simulink model "mux_axi"  (R2023b)
settings: Solver=FixedStepDiscrete  StartTime=0.0  StopTime=1000e-7  RelTol=1e-3
values from neighbouring files (symbols this model uses):
  t_clk = 1/f_clk    (= 1e-08)    [mux_init.m]
libraries: hdlsllib x20, simulink x18
settings Model: DataTypeOverride=Off  Creator=ga92wum  LastModifiedBy=ga92wum
settings SolverCC: AlgebraicLoopSolver=TrustRegion
settings DataIOCC: LimitDataPoints=on  SaveOutput=off  SaveTime=off
settings OptimizationCC: BlockReduction=off  ConditionallyExecuteInputs=off  DefaultParameterBehavior=Inlined  LifeSpan=inf
settings DebuggingCC: AlgebraicLoopMsg=error  SingleTaskRateTransMsg=error  UnconnectedInputMsg=warning  UnconnectedOutputMsg=warning  UnconnectedLineMsg=warning  AllowSymbolicDim=off  StrictBusMsg=ErrorOnBusTreatedAsVector  SFUnexpectedBacktrackingDiag=warning  SFNoUnconditionalDefaultTransitionDiag=warning  SFExecutionAtInitializationDiag=none  ArithmeticOperatorsInVariantConditions=warning
settings HardwareCC: ProdBitPerPointer=32  ProdBitPerSizeT=32  ProdBitPerPtrDiffT=32  ProdLargestAtomicFloat=None  ProdIntDivRoundTo=Undefined  ProdEndianess=Unspecified  ProdWordSize=32  ProdHWDeviceType=ASIC/FPGA->ASIC/FPGA  ProdEqTarget=off
settings ModelReferenceCC: EnableRefExpFcnMdlSchedulingChecks=on
settings SFSimCC: SimUseLocalCustomCode=off  CustomCodeUndefinedFunction=UseInterfaceOnly
settings RTWCC: RTWUseLocalCustomCode=off  DLArmComputeVersion=19.05
settings CodeAppCC: StateflowObjectComments=on
settings GRTTargetCC: TargetLangStandard=C89/C90 (ANSI)
settings ConfigComp: CovScope=ReferencedModels  CovMetricSettings=dw  CovSaveCumulativeToWorkspaceVar=on  CovSaveSingleToWorkspaceVar=on  CovExternalEMLEnable=off  CovSFcnEnable=off

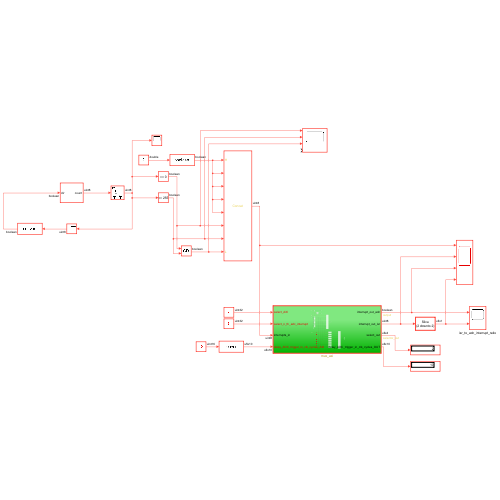
[thumbnail: Simulink's stored preview of the top-level diagram]
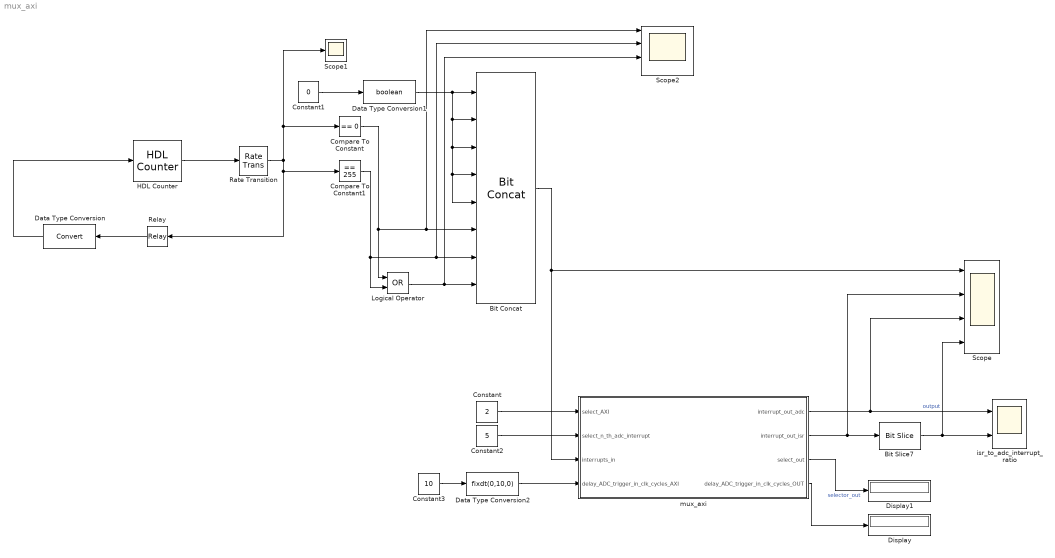
== system mux_axi ==
  Bit Concat : hdlsllib/Logic and Bit Operations/Bit Concat  numInputs=8
  Bit Slice7 : hdlsllib/Logic and Bit Operations/Bit Slice  lidx=2  ridx=2
  Compare To Constant : simulink/Logic and Bit Operations/Compare To Constant  relop===  const=0  OutDataTypeStr=boolean
  Compare To Constant1 : simulink/Logic and Bit Operations/Compare To Constant  relop===  const=255  OutDataTypeStr=boolean
  Constant : Constant  Value=2  OutDataTypeStr=uint32  SampleTime=-1
  Constant1 : Constant  Value=0  SampleTime=-1
  Constant2 : Constant  Value=5  OutDataTypeStr=uint32  SampleTime=-1
  Constant3 : Constant  Value=10  OutDataTypeStr=uint16  SampleTime=-1
  Data Type Conversion : DataTypeConversion  SaturateOnIntegerOverflow=off  RndMeth=Floor
  Data Type Conversion1 : DataTypeConversion  OutDataTypeStr=boolean  SaturateOnIntegerOverflow=off  RndMeth=Floor
  Data Type Conversion2 : DataTypeConversion  OutDataTypeStr=fixdt(0,10,0)  RndMeth=Nearest  SaturateOnIntegerOverflow=off
  Display : Display
  Display1 : Display
  HDL Counter : hdlsllib/Sources/HDL Counter  CountType=Free running  CountInit=0  CountStep=1  CountMax=25  CountFromType=Initial value  CountFrom=0  CountResetPort=off  CountLoadPort=off  CountEnbPort=off  CountDirPort=on  CountHitOutputPort=off  CountDataType=Unsigned  CountWordLen=8  CountFracLen=0  CountSampTime=1
  Logical Operator : Logic  Operator=OR  AllPortsSameDT=off  OutDataTypeStr=boolean
  Rate Transition : RateTransition  OutPortSampleTime=t_clk
  Relay : Relay  OnSwitchValue=256  OffSwitchValue=0  OnOutputValue=0  OffOutputValue=1
  Scope : Scope  NumInputPorts=4
  Scope1 : Scope
  Scope2 : Scope  NumInputPorts=4
  isr_to_adc_interrupt_ratio : Scope  NumInputPorts=2
  mux_axi : Subsystem  TreatAsAtomicUnit=on
  wires:
  mux_axi/1(interrupt_out_adc) -> Scope/3, isr_to_adc_interrupt_ratio/1  "output"
  Constant/1 -> mux_axi/1(select_AXI)
  Bit Concat/1 -> mux_axi/3(interrupts_in), Scope/1
  Constant2/1 -> mux_axi/2(select_n_th_adc_interrupt)
  mux_axi/2(interrupt_out_isr) -> Scope/2, Bit Slice7/1
  HDL Counter/1 -> Rate Transition/1
  Rate Transition/1 -> Compare To Constant/1, Scope1/1, Compare To Constant1/1, Relay/1
  Relay/1 -> Data Type Conversion/1
  Data Type Conversion/1 -> HDL Counter/1
  Compare To Constant/1 -> Scope2/1, Bit Concat/6, Logical Operator/1
  Compare To Constant1/1 -> Bit Concat/7, Scope2/2, Logical Operator/2
  Logical Operator/1 -> Bit Concat/8, Scope2/3
  Constant1/1 -> Data Type Conversion1/1
  Data Type Conversion1/1 -> Bit Concat/5, Bit Concat/4, Bit Concat/3, Bit Concat/2, Bit Concat/1
  Constant3/1 -> Data Type Conversion2/1
  mux_axi/4(delay_ADC_trigger_in_clk_cycles_OUT) -> Display/1
  Data Type Conversion2/1 -> mux_axi/4(delay_ADC_trigger_in_clk_cycles_AXI)
  Bit Slice7/1 -> Scope/4, isr_to_adc_interrupt_ratio/2
  mux_axi/3(select_out) -> Display1/1  "selector_out"

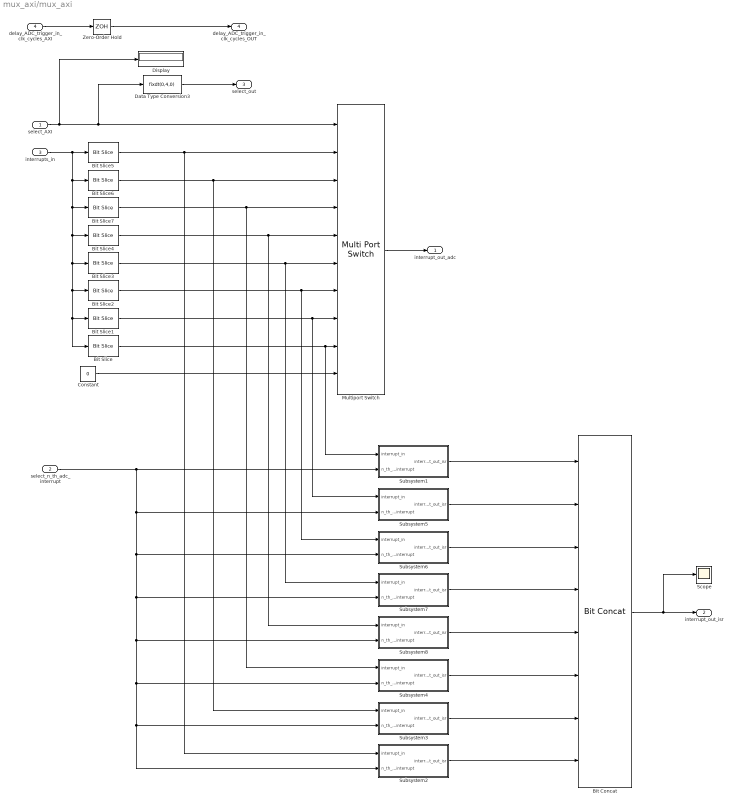
== system mux_axi/mux_axi ==
  select_AXI : Inport
  select_n_th_adc_interrupt : Inport  Port=2
  interrupts_in : Inport  Port=3  OutDataTypeStr=uint8
  delay_ADC_trigger_in_clk_cycles_AXI : Inport  Port=4  OutDataTypeStr=fixdt(0,10,0)
  Bit Concat : hdlsllib/Logic and Bit Operations/Bit Concat  numInputs=8
  Bit Slice : hdlsllib/Logic and Bit Operations/Bit Slice  lidx=7  ridx=7
  Bit Slice1 : hdlsllib/Logic and Bit Operations/Bit Slice  lidx=6  ridx=6
  Bit Slice2 : hdlsllib/Logic and Bit Operations/Bit Slice  lidx=5  ridx=5
  Bit Slice3 : hdlsllib/Logic and Bit Operations/Bit Slice  lidx=4  ridx=4
  Bit Slice4 : hdlsllib/Logic and Bit Operations/Bit Slice  lidx=3  ridx=3
  Bit Slice5 : hdlsllib/Logic and Bit Operations/Bit Slice  lidx=0  ridx=0
  Bit Slice6 : hdlsllib/Logic and Bit Operations/Bit Slice  lidx=1  ridx=1
  Bit Slice7 : hdlsllib/Logic and Bit Operations/Bit Slice  lidx=2  ridx=2
  Constant : Constant  Value=0  OutDataTypeStr=boolean  SampleTime=t_clk
  Data Type Conversion3 : DataTypeConversion  OutDataTypeStr=fixdt(0,4,0)  SaturateOnIntegerOverflow=off  RndMeth=Floor
  Display : Display
  Multiport Switch : MultiPortSwitch  DataPortOrder=Zero-based contiguous  Inputs=8  DataPortForDefault=Additional data port  zeroidx=on  SaturateOnIntegerOverflow=off  InputSameDT=off
  Scope : Scope
  Subsystem1 : Subsystem
  Subsystem2 : Subsystem
  Subsystem3 : Subsystem
  Subsystem4 : Subsystem
  Subsystem5 : Subsystem
  Subsystem6 : Subsystem
  Subsystem7 : Subsystem
  Subsystem8 : Subsystem
  Zero-Order Hold : ZeroOrderHold  SampleTime=-1
  interrupt_out_adc : Outport  OutDataTypeStr=boolean  VectorParamsAs1DForOutWhenUnconnected=off
  interrupt_out_isr : Outport  Port=2  VectorParamsAs1DForOutWhenUnconnected=off
  select_out : Outport  Port=3  VectorParamsAs1DForOutWhenUnconnected=off
  delay_ADC_trigger_in_clk_cycles_OUT : Outport  Port=4  VectorParamsAs1DForOutWhenUnconnected=off
  wires:
  Bit Slice3/1 -> Subsystem7/1(interrupt_in), Multiport Switch/6
  Bit Slice4/1 -> Multiport Switch/5, Subsystem8/1(interrupt_in)
  Bit Slice7/1 -> Multiport Switch/4, Subsystem4/1(interrupt_in)
  Bit Slice6/1 -> Multiport Switch/3, Subsystem3/1(interrupt_in)
  Bit Slice5/1 -> Multiport Switch/2, Subsystem2/1(interrupt_in)
  Bit Slice/1 -> Subsystem1/1(interrupt_in), Multiport Switch/9
  Constant/1 -> Multiport Switch/10
  Bit Slice1/1 -> Subsystem5/1(interrupt_in), Multiport Switch/8
  Data Type Conversion3/1 -> select_out/1
  interrupts_in/1 -> Bit Slice/1, Bit Slice1/1, Bit Slice2/1, Bit Slice3/1, Bit Slice4/1, Bit Slice7/1, Bit Slice6/1, Bit Slice5/1
  select_n_th_adc_interrupt/1 -> Subsystem1/2(n_th_adc_interrupt), Subsystem5/2(n_th_adc_interrupt), Subsystem6/2(n_th_adc_interrupt), Subsystem7/2(n_th_adc_interrupt), Subsystem8/2(n_th_adc_interrupt), Subsystem4/2(n_th_adc_interrupt), Subsystem2/2(n_th_adc_interrupt), Subsystem3/2(n_th_adc_interrupt)
  Bit Concat/1 -> Scope/1, interrupt_out_isr/1
  Multiport Switch/1 -> interrupt_out_adc/1
  select_AXI/1 -> Display/1, Data Type Conversion3/1, Multiport Switch/1
  delay_ADC_trigger_in_clk_cycles_AXI/1 -> Zero-Order Hold/1
  Zero-Order Hold/1 -> delay_ADC_trigger_in_clk_cycles_OUT/1
  Subsystem1/1(interrupt_out_isr) -> Bit Concat/1
  Subsystem3/1(interrupt_out_isr) -> Bit Concat/7
  Subsystem2/1(interrupt_out_isr) -> Bit Concat/8
  Subsystem4/1(interrupt_out_isr) -> Bit Concat/6
  Subsystem8/1(interrupt_out_isr) -> Bit Concat/5
  Subsystem7/1(interrupt_out_isr) -> Bit Concat/4
  Subsystem6/1(interrupt_out_isr) -> Bit Concat/3
  Subsystem5/1(interrupt_out_isr) -> Bit Concat/2
  Bit Slice2/1 -> Subsystem6/1(interrupt_in), Multiport Switch/7

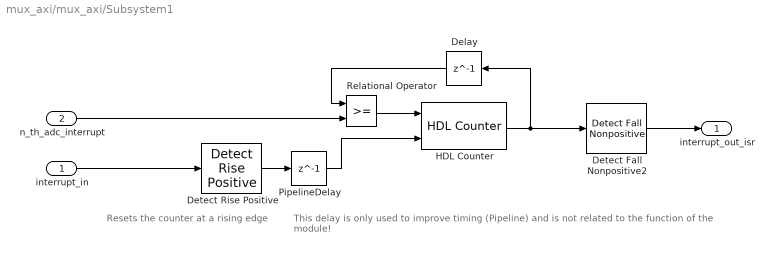
== system mux_axi/mux_axi/Subsystem1 ==
  note: This delay is only used to improve timing (Pipeline) and is not related to the function of the module!
  note: Resets the counter at a rising edge
  interrupt_in : Inport
  n_th_adc_interrupt : Inport  Port=2
  Delay : Delay  DelayLength=1
  Detect Fall Nonpositive2 : simulink/Logic and Bit Operations/Detect Fall Nonpositive  vinit=0  OutDataTypeStr=boolean
  Detect Rise Positive : simulink/Logic and Bit Operations/Detect Rise Positive  vinit=0  OutDataTypeStr=boolean
  HDL Counter : hdlsllib/Sources/HDL Counter  CountType=Free running  CountInit=0  CountStep=1  CountMax=25  CountFromType=Initial value  CountFrom=0  CountResetPort=on  CountLoadPort=off  CountEnbPort=on  CountDirPort=off  CountHitOutputPort=off  CountDataType=Unsigned  CountWordLen=8  CountFracLen=0  CountSampTime=-1
  PipelineDelay : Delay  DelayLength=1
  Relational Operator : RelationalOperator  OutDataTypeStr=boolean  RndMeth=Simplest  InputSameDT=off
  interrupt_out_isr : Outport
  wires:
  Detect Rise Positive/1 -> PipelineDelay/1
  interrupt_in/1 -> Detect Rise Positive/1
  n_th_adc_interrupt/1 -> Relational Operator/2
  PipelineDelay/1 -> HDL Counter/2
  Relational Operator/1 -> HDL Counter/1
  HDL Counter/1 -> Delay/1, Detect Fall Nonpositive2/1
  Delay/1 -> Relational Operator/1
  Detect Fall Nonpositive2/1 -> interrupt_out_isr/1

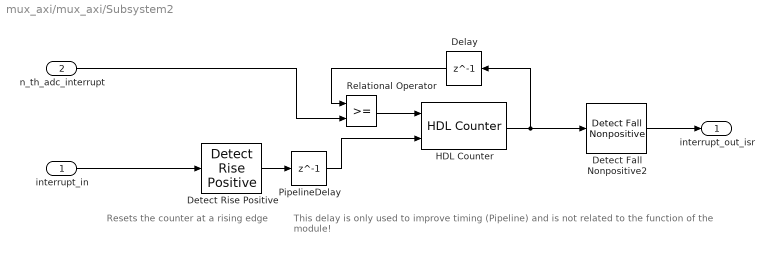
== system mux_axi/mux_axi/Subsystem2 ==
  note: Resets the counter at a rising edge
  note: This delay is only used to improve timing (Pipeline) and is not related to the function of the module!
  interrupt_in : Inport
  n_th_adc_interrupt : Inport  Port=2
  Delay : Delay  DelayLength=1
  Detect Fall Nonpositive2 : simulink/Logic and Bit Operations/Detect Fall Nonpositive  vinit=0  OutDataTypeStr=boolean
  Detect Rise Positive : simulink/Logic and Bit Operations/Detect Rise Positive  vinit=0  OutDataTypeStr=boolean
  HDL Counter : hdlsllib/Sources/HDL Counter  CountType=Free running  CountInit=0  CountStep=1  CountMax=25  CountFromType=Initial value  CountFrom=0  CountResetPort=on  CountLoadPort=off  CountEnbPort=on  CountDirPort=off  CountHitOutputPort=off  CountDataType=Unsigned  CountWordLen=8  CountFracLen=0  CountSampTime=-1
  PipelineDelay : Delay  DelayLength=1
  Relational Operator : RelationalOperator  OutDataTypeStr=boolean  RndMeth=Simplest  InputSameDT=off
  interrupt_out_isr : Outport
  wires:
  Detect Fall Nonpositive2/1 -> interrupt_out_isr/1
  Delay/1 -> Relational Operator/1
  HDL Counter/1 -> Detect Fall Nonpositive2/1, Delay/1
  Relational Operator/1 -> HDL Counter/1
  PipelineDelay/1 -> HDL Counter/2
  n_th_adc_interrupt/1 -> Relational Operator/2
  interrupt_in/1 -> Detect Rise Positive/1
  Detect Rise Positive/1 -> PipelineDelay/1

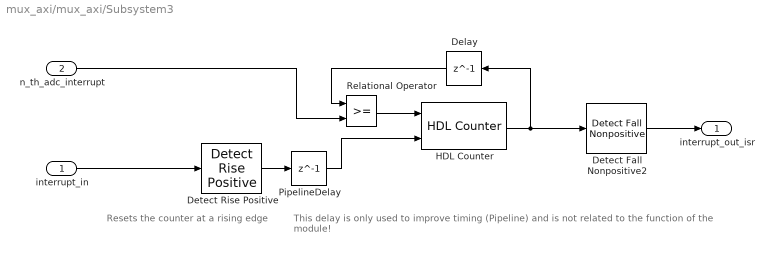
== system mux_axi/mux_axi/Subsystem3 ==
  note: This delay is only used to improve timing (Pipeline) and is not related to the function of the module!
  note: Resets the counter at a rising edge
  interrupt_in : Inport
  n_th_adc_interrupt : Inport  Port=2
  Delay : Delay  DelayLength=1
  Detect Fall Nonpositive2 : simulink/Logic and Bit Operations/Detect Fall Nonpositive  vinit=0  OutDataTypeStr=boolean
  Detect Rise Positive : simulink/Logic and Bit Operations/Detect Rise Positive  vinit=0  OutDataTypeStr=boolean
  HDL Counter : hdlsllib/Sources/HDL Counter  CountType=Free running  CountInit=0  CountStep=1  CountMax=25  CountFromType=Initial value  CountFrom=0  CountResetPort=on  CountLoadPort=off  CountEnbPort=on  CountDirPort=off  CountHitOutputPort=off  CountDataType=Unsigned  CountWordLen=8  CountFracLen=0  CountSampTime=-1
  PipelineDelay : Delay  DelayLength=1
  Relational Operator : RelationalOperator  OutDataTypeStr=boolean  RndMeth=Simplest  InputSameDT=off
  interrupt_out_isr : Outport
  wires:
  Detect Rise Positive/1 -> PipelineDelay/1
  interrupt_in/1 -> Detect Rise Positive/1
  n_th_adc_interrupt/1 -> Relational Operator/2
  PipelineDelay/1 -> HDL Counter/2
  Relational Operator/1 -> HDL Counter/1
  HDL Counter/1 -> Delay/1, Detect Fall Nonpositive2/1
  Delay/1 -> Relational Operator/1
  Detect Fall Nonpositive2/1 -> interrupt_out_isr/1

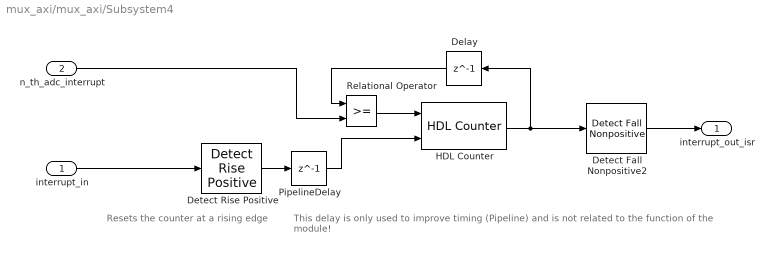
== system mux_axi/mux_axi/Subsystem4 ==
  note: Resets the counter at a rising edge
  note: This delay is only used to improve timing (Pipeline) and is not related to the function of the module!
  interrupt_in : Inport
  n_th_adc_interrupt : Inport  Port=2
  Delay : Delay  DelayLength=1
  Detect Fall Nonpositive2 : simulink/Logic and Bit Operations/Detect Fall Nonpositive  vinit=0  OutDataTypeStr=boolean
  Detect Rise Positive : simulink/Logic and Bit Operations/Detect Rise Positive  vinit=0  OutDataTypeStr=boolean
  HDL Counter : hdlsllib/Sources/HDL Counter  CountType=Free running  CountInit=0  CountStep=1  CountMax=25  CountFromType=Initial value  CountFrom=0  CountResetPort=on  CountLoadPort=off  CountEnbPort=on  CountDirPort=off  CountHitOutputPort=off  CountDataType=Unsigned  CountWordLen=8  CountFracLen=0  CountSampTime=-1
  PipelineDelay : Delay  DelayLength=1
  Relational Operator : RelationalOperator  OutDataTypeStr=boolean  RndMeth=Simplest  InputSameDT=off
  interrupt_out_isr : Outport
  wires:
  Detect Fall Nonpositive2/1 -> interrupt_out_isr/1
  Delay/1 -> Relational Operator/1
  HDL Counter/1 -> Detect Fall Nonpositive2/1, Delay/1
  Relational Operator/1 -> HDL Counter/1
  PipelineDelay/1 -> HDL Counter/2
  n_th_adc_interrupt/1 -> Relational Operator/2
  interrupt_in/1 -> Detect Rise Positive/1
  Detect Rise Positive/1 -> PipelineDelay/1

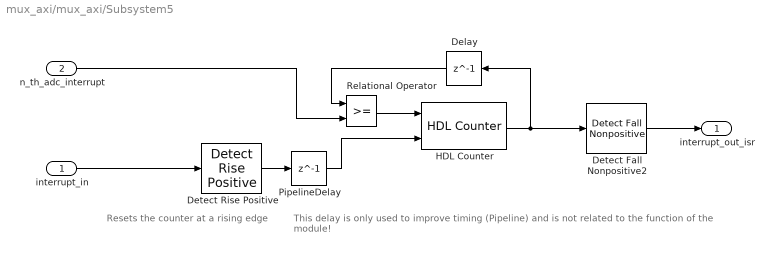
== system mux_axi/mux_axi/Subsystem5 ==
  note: Resets the counter at a rising edge
  note: This delay is only used to improve timing (Pipeline) and is not related to the function of the module!
  interrupt_in : Inport
  n_th_adc_interrupt : Inport  Port=2
  Delay : Delay  DelayLength=1
  Detect Fall Nonpositive2 : simulink/Logic and Bit Operations/Detect Fall Nonpositive  vinit=0  OutDataTypeStr=boolean
  Detect Rise Positive : simulink/Logic and Bit Operations/Detect Rise Positive  vinit=0  OutDataTypeStr=boolean
  HDL Counter : hdlsllib/Sources/HDL Counter  CountType=Free running  CountInit=0  CountStep=1  CountMax=25  CountFromType=Initial value  CountFrom=0  CountResetPort=on  CountLoadPort=off  CountEnbPort=on  CountDirPort=off  CountHitOutputPort=off  CountDataType=Unsigned  CountWordLen=8  CountFracLen=0  CountSampTime=-1
  PipelineDelay : Delay  DelayLength=1
  Relational Operator : RelationalOperator  OutDataTypeStr=boolean  RndMeth=Simplest  InputSameDT=off
  interrupt_out_isr : Outport
  wires:
  Detect Fall Nonpositive2/1 -> interrupt_out_isr/1
  Delay/1 -> Relational Operator/1
  HDL Counter/1 -> Detect Fall Nonpositive2/1, Delay/1
  Relational Operator/1 -> HDL Counter/1
  PipelineDelay/1 -> HDL Counter/2
  n_th_adc_interrupt/1 -> Relational Operator/2
  interrupt_in/1 -> Detect Rise Positive/1
  Detect Rise Positive/1 -> PipelineDelay/1

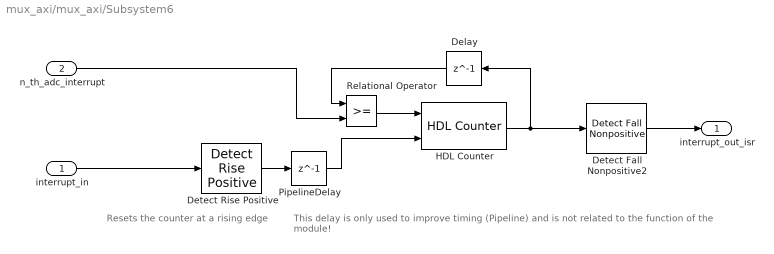
== system mux_axi/mux_axi/Subsystem6 ==
  note: This delay is only used to improve timing (Pipeline) and is not related to the function of the module!
  note: Resets the counter at a rising edge
  interrupt_in : Inport
  n_th_adc_interrupt : Inport  Port=2
  Delay : Delay  DelayLength=1
  Detect Fall Nonpositive2 : simulink/Logic and Bit Operations/Detect Fall Nonpositive  vinit=0  OutDataTypeStr=boolean
  Detect Rise Positive : simulink/Logic and Bit Operations/Detect Rise Positive  vinit=0  OutDataTypeStr=boolean
  HDL Counter : hdlsllib/Sources/HDL Counter  CountType=Free running  CountInit=0  CountStep=1  CountMax=25  CountFromType=Initial value  CountFrom=0  CountResetPort=on  CountLoadPort=off  CountEnbPort=on  CountDirPort=off  CountHitOutputPort=off  CountDataType=Unsigned  CountWordLen=8  CountFracLen=0  CountSampTime=-1
  PipelineDelay : Delay  DelayLength=1
  Relational Operator : RelationalOperator  OutDataTypeStr=boolean  RndMeth=Simplest  InputSameDT=off
  interrupt_out_isr : Outport
  wires:
  Detect Rise Positive/1 -> PipelineDelay/1
  interrupt_in/1 -> Detect Rise Positive/1
  n_th_adc_interrupt/1 -> Relational Operator/2
  PipelineDelay/1 -> HDL Counter/2
  Relational Operator/1 -> HDL Counter/1
  HDL Counter/1 -> Delay/1, Detect Fall Nonpositive2/1
  Delay/1 -> Relational Operator/1
  Detect Fall Nonpositive2/1 -> interrupt_out_isr/1

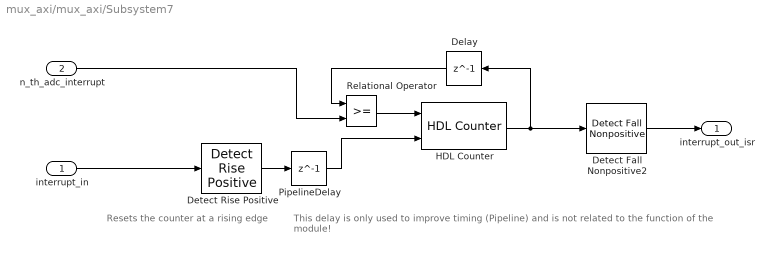
== system mux_axi/mux_axi/Subsystem7 ==
  note: Resets the counter at a rising edge
  note: This delay is only used to improve timing (Pipeline) and is not related to the function of the module!
  interrupt_in : Inport
  n_th_adc_interrupt : Inport  Port=2
  Delay : Delay  DelayLength=1
  Detect Fall Nonpositive2 : simulink/Logic and Bit Operations/Detect Fall Nonpositive  vinit=0  OutDataTypeStr=boolean
  Detect Rise Positive : simulink/Logic and Bit Operations/Detect Rise Positive  vinit=0  OutDataTypeStr=boolean
  HDL Counter : hdlsllib/Sources/HDL Counter  CountType=Free running  CountInit=0  CountStep=1  CountMax=25  CountFromType=Initial value  CountFrom=0  CountResetPort=on  CountLoadPort=off  CountEnbPort=on  CountDirPort=off  CountHitOutputPort=off  CountDataType=Unsigned  CountWordLen=8  CountFracLen=0  CountSampTime=-1
  PipelineDelay : Delay  DelayLength=1
  Relational Operator : RelationalOperator  OutDataTypeStr=boolean  RndMeth=Simplest  InputSameDT=off
  interrupt_out_isr : Outport
  wires:
  Detect Fall Nonpositive2/1 -> interrupt_out_isr/1
  Delay/1 -> Relational Operator/1
  HDL Counter/1 -> Detect Fall Nonpositive2/1, Delay/1
  Relational Operator/1 -> HDL Counter/1
  PipelineDelay/1 -> HDL Counter/2
  n_th_adc_interrupt/1 -> Relational Operator/2
  interrupt_in/1 -> Detect Rise Positive/1
  Detect Rise Positive/1 -> PipelineDelay/1

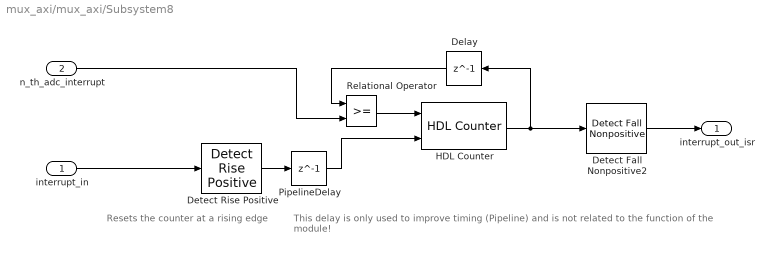
== system mux_axi/mux_axi/Subsystem8 ==
  note: This delay is only used to improve timing (Pipeline) and is not related to the function of the module!
  note: Resets the counter at a rising edge
  interrupt_in : Inport
  n_th_adc_interrupt : Inport  Port=2
  Delay : Delay  DelayLength=1
  Detect Fall Nonpositive2 : simulink/Logic and Bit Operations/Detect Fall Nonpositive  vinit=0  OutDataTypeStr=boolean
  Detect Rise Positive : simulink/Logic and Bit Operations/Detect Rise Positive  vinit=0  OutDataTypeStr=boolean
  HDL Counter : hdlsllib/Sources/HDL Counter  CountType=Free running  CountInit=0  CountStep=1  CountMax=25  CountFromType=Initial value  CountFrom=0  CountResetPort=on  CountLoadPort=off  CountEnbPort=on  CountDirPort=off  CountHitOutputPort=off  CountDataType=Unsigned  CountWordLen=8  CountFracLen=0  CountSampTime=-1
  PipelineDelay : Delay  DelayLength=1
  Relational Operator : RelationalOperator  OutDataTypeStr=boolean  RndMeth=Simplest  InputSameDT=off
  interrupt_out_isr : Outport
  wires:
  Detect Rise Positive/1 -> PipelineDelay/1
  interrupt_in/1 -> Detect Rise Positive/1
  n_th_adc_interrupt/1 -> Relational Operator/2
  PipelineDelay/1 -> HDL Counter/2
  Relational Operator/1 -> HDL Counter/1
  HDL Counter/1 -> Delay/1, Detect Fall Nonpositive2/1
  Delay/1 -> Relational Operator/1
  Detect Fall Nonpositive2/1 -> interrupt_out_isr/1
